simulink model "open_loop"  (Simulink 7.9)
settings: Solver=FixedStepDiscrete  StartTime=0.0  StopTime=tend  FixedStep=params.th  MaxStep=0.01  RelTol=1e-6  AbsTol=1e-3
values from neighbouring files (symbols this model uses):
  delta_pot = 0    [check.m]    (also in ctrl_design.m; plant_info.m)
  delta_vel = 0    [check.m]    (also in ctrl_design.m; plant_info.m = 1e-05)
undefined symbols (not defined in the file or in its folder): params
settings Model: Creator=puri  LastModifiedBy=Jorge
settings CodeAppCC: CustomSymbolStrType=$N$R$M_T
settings GRTTargetCC: CodeReplacementLibrary=None  CPPClassGenCompliant=on

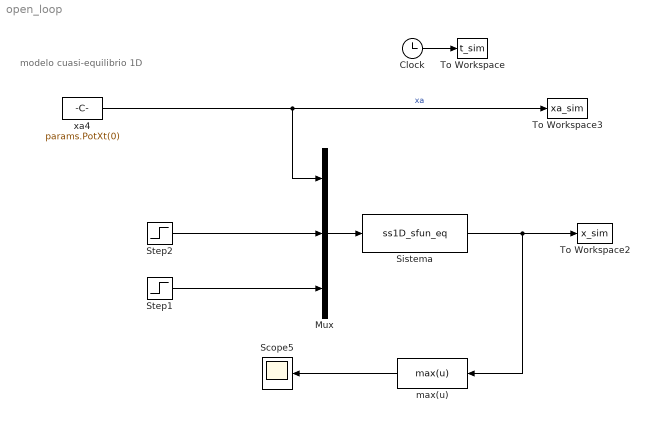
== system open_loop ==
  note: modelo cuasi-equilibrio 1D
  Clock : Clock
  Mux : Mux  Inputs=3
  Scope5 : Scope
      settings: TimeRange=4  YMin=4942.75  YMax=4948  SaveName=ScopeData5
  Sistema : S-Function  FunctionName=ss1D_sfun_eq  EnableBusSupport=off
      settings: DeleteFcn=shh = get(0,'ShowHiddenHandles');set(0,'ShowHiddenHandles','on');if ~isempty(findobj('type','figure','name','dblcart1 Animation'));close('dblcart1 Animation'); end;set(0,'ShowHiddenHandles',shh);
  Step1 : Step  Time=0  Before=params.v(0)  After=params.v(0) + delta_vel  SampleTime=0
  Step2 : Step  Time=0  Before=params.Pot(0)  After=params.Pot(0) + delta_pot  SampleTime=0
  To Workspace : ToWorkspace  VariableName=t_sim  SampleTime=-1
  To Workspace2 : ToWorkspace  VariableName=x_sim  SampleTime=-1
  To Workspace3 : ToWorkspace  VariableName=xa_sim  SampleTime=-1
  max(u) : MATLABFcn  MATLABFcn=max(u)
  xa4 : Constant  Value=params.PotXt(0)
  wires:
  Mux/1 -> Sistema/1
  Sistema/1 -> To Workspace2/1, max(u)/1
  xa4/1 -> Mux/1, To Workspace3/1  "xa"
  Clock/1 -> To Workspace/1
  max(u)/1 -> Scope5/1
  Step1/1 -> Mux/3
  Step2/1 -> Mux/2
